simulink library "slrt2levelinverterlib"  (R2022b)
settings: Solver=VariableStepAuto  StartTime=0.0  StopTime=10.0  RelTol=1e-3
libraries: simulink x40, slrthdlutillib x12, hdlsllib x3
settings Model: Creator=chrisz  LastModifiedBy=chrisz
settings ModelReferenceCC: EnableRefExpFcnMdlSchedulingChecks=on
settings RTWCC: PlatformDefinition=Embedded Code

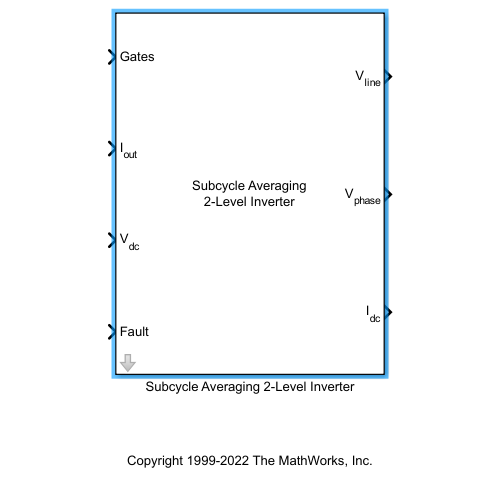
[thumbnail: Simulink's stored preview of the top-level diagram]
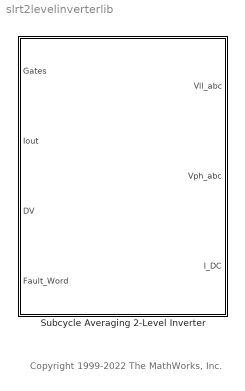
== system slrt2levelinverterlib ==
  note: Copyright 1999-2022 The MathWorks, Inc.
  "Subcycle Averaging 2-Level Inverter " : Subsystem  mask(Subcycle Averaging 2-level Inverter){rSwitch=0.1, vfSwitch=0.8, rDiode=0.2, vfDiode=0.6, rSnub=10000, ts_Model=1e-6, ts_FPGA=5e-9}
      mask prompts: rSwitch "Switch Resistance (Ohms)"; vfSwitch "Switch Forward Voltage (V)"; rDiode "Diode Resistance (Ohms)"; vfDiode "Diode Forward Voltage (V)"; rSnub "Snubber Resistance (Ohms)"; ts_Model "Model Time Step (s)"; ts_FPGA "FPGA Time Step (s)"
      mask help:
      | 2 level inverter with subcycle averaging that is meant for implementation of real-time models.  This model simulates FPGA clock level operations and is not suited for desktop simulation other than for validating the real-time model is accurate.  It should primarily be used when generating HDL for real-time systems. Use standard converter models and blocks for desktop simulation.
      |
      | Model time step should be 1/10 of switching frequency to capture accurate switching waveforms. FPGA time step should be the fastest time step you can run your HIL FPGA at.
      mask DialogControl ParameterGroupVar Prompt: Physical Parameters
      mask DialogControl Container3 Prompt: Simulation Parameters
      mask Display:
      | disp('Subcycle Averaging\n2-Level Inverter');
      | port_label('input',1,'Gates');
      | port_label('input',2,'I_o_u_t','texmode','on');
      | port_label('input',3,'V_d_c','texmode','on');
      | port_label('input',4,'Fault');
      | port_label('output',1,'V_l_i_n_e','texmode','on');
      | port_label('output',2,'V_p_h_a_s_e','texmode','on');
      | port_label('output',3,'I_d_c','texmode','on');

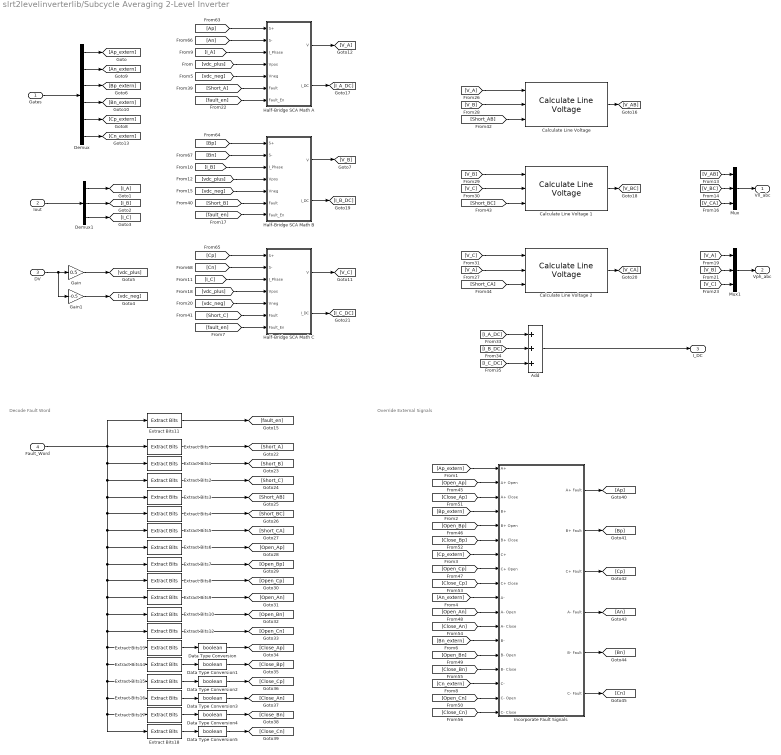
== system slrt2levelinverterlib/Subcycle Averaging 2-Level Inverter  ==
  note: Override External Signals
  note: Decode Fault Word
  Gates : Inport
  Iout : Inport  Port=2
  DV : Inport  Port=3
  Fault_Word : Inport  Port=4
  Add : Sum  Inputs=+++
  "Calculate Line Voltage " : slrthdlutillib/Calculate Line Voltage 
  Calculate Line Voltage 1 : slrthdlutillib/Calculate Line Voltage 
  Calculate Line Voltage 2 : slrthdlutillib/Calculate Line Voltage 
  Data Type Conversion{,1..5} (6 alike) : DataTypeConversion  OutDataTypeStr=boolean  SaturateOnIntegerOverflow=off  RndMeth=Floor
  Demux : Demux  Outputs=6
  Demux1 : Demux  Outputs=3
  Extract Bits : simulink/Logic and Bit Operations/Extract Bits  bitsToExtract=Range of bits  numBits=8  bitIdxRange=[0]  outScalingMode=Treat bit field as an integer
  Extract Bits1 : simulink/Logic and Bit Operations/Extract Bits  bitsToExtract=Range of bits  numBits=8  bitIdxRange=1  outScalingMode=Treat bit field as an integer
  Extract Bits10 : simulink/Logic and Bit Operations/Extract Bits  bitsToExtract=Range of bits  numBits=8  bitIdxRange=10  outScalingMode=Treat bit field as an integer
  Extract Bits11 : simulink/Logic and Bit Operations/Extract Bits  bitsToExtract=Range of bits  numBits=8  bitIdxRange=[31]  outScalingMode=Treat bit field as an integer
  Extract Bits12 : simulink/Logic and Bit Operations/Extract Bits  bitsToExtract=Range of bits  numBits=8  bitIdxRange=11  outScalingMode=Treat bit field as an integer
  Extract Bits13 : simulink/Logic and Bit Operations/Extract Bits  bitsToExtract=Range of bits  numBits=8  bitIdxRange=12  outScalingMode=Treat bit field as an integer
  Extract Bits14 : simulink/Logic and Bit Operations/Extract Bits  bitsToExtract=Range of bits  numBits=8  bitIdxRange=13  outScalingMode=Treat bit field as an integer
  Extract Bits15 : simulink/Logic and Bit Operations/Extract Bits  bitsToExtract=Range of bits  numBits=8  bitIdxRange=14  outScalingMode=Treat bit field as an integer
  Extract Bits16 : simulink/Logic and Bit Operations/Extract Bits  bitsToExtract=Range of bits  numBits=8  bitIdxRange=15  outScalingMode=Treat bit field as an integer
  Extract Bits17 : simulink/Logic and Bit Operations/Extract Bits  bitsToExtract=Range of bits  numBits=8  bitIdxRange=16  outScalingMode=Treat bit field as an integer
  Extract Bits18 : simulink/Logic and Bit Operations/Extract Bits  bitsToExtract=Range of bits  numBits=8  bitIdxRange=17  outScalingMode=Treat bit field as an integer
  Extract Bits2 : simulink/Logic and Bit Operations/Extract Bits  bitsToExtract=Range of bits  numBits=8  bitIdxRange=2  outScalingMode=Treat bit field as an integer
  Extract Bits3 : simulink/Logic and Bit Operations/Extract Bits  bitsToExtract=Range of bits  numBits=8  bitIdxRange=3  outScalingMode=Treat bit field as an integer
  Extract Bits4 : simulink/Logic and Bit Operations/Extract Bits  bitsToExtract=Range of bits  numBits=8  bitIdxRange=4  outScalingMode=Treat bit field as an integer
  Extract Bits5 : simulink/Logic and Bit Operations/Extract Bits  bitsToExtract=Range of bits  numBits=8  bitIdxRange=5  outScalingMode=Treat bit field as an integer
  Extract Bits6 : simulink/Logic and Bit Operations/Extract Bits  bitsToExtract=Range of bits  numBits=8  bitIdxRange=6  outScalingMode=Treat bit field as an integer
  Extract Bits7 : simulink/Logic and Bit Operations/Extract Bits  bitsToExtract=Range of bits  numBits=8  bitIdxRange=7  outScalingMode=Treat bit field as an integer
  Extract Bits8 : simulink/Logic and Bit Operations/Extract Bits  bitsToExtract=Range of bits  numBits=8  bitIdxRange=8  outScalingMode=Treat bit field as an integer
  Extract Bits9 : simulink/Logic and Bit Operations/Extract Bits  bitsToExtract=Range of bits  numBits=8  bitIdxRange=9  outScalingMode=Treat bit field as an integer
  Gain : Gain  Gain=0.5
  Gain1 : Gain  Gain=-0.5
  Half-Bridge SCA Math A : Subsystem
  Half-Bridge SCA Math B : Subsystem
  Half-Bridge SCA Math C : Subsystem
  Incorporate Fault Signals : Subsystem
  Mux : Mux  Inputs=3
  Mux1 : Mux  Inputs=3
  Vll_abc : Outport  OutDataTypeStr=single  VectorParamsAs1DForOutWhenUnconnected=off
  Vph_abc : Outport  Port=2  OutDataTypeStr=single  VectorParamsAs1DForOutWhenUnconnected=off
  I_DC : Outport  Port=3  OutDataTypeStr=single  VectorParamsAs1DForOutWhenUnconnected=off
  wires:
  Gates/1 -> Demux/1
  Demux/1 -> [Ap_extern]
  Demux/3 -> [Bp_extern]
  Demux/5 -> [Cp_extern]
  Half-Bridge SCA Math A/1(V) -> [V_A]
  [V_B] -> "Calculate Line Voltage "/2
  [V_A] -> "Calculate Line Voltage "/1
  Extract Bits9/1 -> [Open_An]
  Extract Bits12/1 -> [Open_Cn]
  [Ap_extern] -> Incorporate Fault Signals/1(A+)
  Incorporate Fault Signals/6(C- Fault) -> [Cn]
  [Open_Cn] -> Incorporate Fault Signals/17(C- Open)
  Incorporate Fault Signals/2(B+ Fault) -> [Bp]
  [Cn_extern] -> Incorporate Fault Signals/16(C-)
  [Close_Bn] -> Incorporate Fault Signals/15(B- Close)
  Incorporate Fault Signals/5(B- Fault) -> [Bn]
  Extract Bits7/1 -> [Open_Bp]
  [Bp_extern] -> Incorporate Fault Signals/4(B+)
  [Close_Cn] -> Incorporate Fault Signals/18(C- Close)
  [Close_Bp] -> Incorporate Fault Signals/6(B+ Close)
  [Open_Bp] -> Incorporate Fault Signals/5(B+ Open)
  [Bn_extern] -> Incorporate Fault Signals/13(B-)
  [Close_An] -> Incorporate Fault Signals/12(A- Close)
  [An_extern] -> Incorporate Fault Signals/10(A-)
  Fault_Word/1 -> Extract Bits11/1, Extract Bits/1, Extract Bits1/1, Extract Bits2/1, Extract Bits3/1, Extract Bits4/1, Extract Bits5/1, Extract Bits6/1, Extract Bits7/1, Extract Bits8/1, Extract Bits9/1, Extract Bits10/1, Extract Bits12/1, Extract Bits13/1, Extract Bits14/1, Extract Bits15/1, Extract Bits16/1, Extract Bits18/1, Extract Bits17/1
  Extract Bits6/1 -> [Open_Ap]
  [Open_Ap] -> Incorporate Fault Signals/2(A+ Open)
  Extract Bits8/1 -> [Open_Cp]
  Extract Bits17/1 -> Data Type Conversion4/1
  [Cp_extern] -> Incorporate Fault Signals/7(C+)
  Extract Bits5/1 -> [Short_CA]
  Extract Bits14/1 -> Data Type Conversion1/1
  Extract Bits1/1 -> [Short_B]
  Extract Bits13/1 -> Data Type Conversion/1
  Extract Bits10/1 -> [Open_Bn]
  Incorporate Fault Signals/4(A- Fault) -> [An]
  [Close_Ap] -> Incorporate Fault Signals/3(A+ Close)
  [Open_Cp] -> Incorporate Fault Signals/8(C+ Open)
  Incorporate Fault Signals/1(A+ Fault) -> [Ap]
  Extract Bits4/1 -> [Short_BC]
  Extract Bits18/1 -> Data Type Conversion5/1
  Extract Bits3/1 -> [Short_AB]
  [Open_Bn] -> Incorporate Fault Signals/14(B- Open)
  Extract Bits2/1 -> [Short_C]
  [Open_An] -> Incorporate Fault Signals/11(A- Open)
  Extract Bits15/1 -> Data Type Conversion2/1
  Extract Bits/1 -> [Short_A]
  Incorporate Fault Signals/3(C+ Fault) -> [Cp]
  [Close_Cp] -> Incorporate Fault Signals/9(C+ Close)
  Extract Bits16/1 -> Data Type Conversion3/1
  Iout/1 -> Demux1/1
  Demux1/1 -> [I_A]
  Demux1/2 -> [I_B]
  Demux1/3 -> [I_C]
  [Ap] -> Half-Bridge SCA Math A/1(S+)
  [I_A] -> Half-Bridge SCA Math A/3(I_Phase)
  [An] -> Half-Bridge SCA Math A/2(S-)
  [vdc_plus] -> Half-Bridge SCA Math A/4(Vpos)
  [vdc_neg] -> Half-Bridge SCA Math A/5(Vneg)
  [Short_A] -> Half-Bridge SCA Math A/6(Fault)
  [Bp] -> Half-Bridge SCA Math B/1(S+)
  [Bn] -> Half-Bridge SCA Math B/2(S-)
  [I_B] -> Half-Bridge SCA Math B/3(I_Phase)
  [vdc_plus] -> Half-Bridge SCA Math B/4(Vpos)
  [vdc_neg] -> Half-Bridge SCA Math B/5(Vneg)
  [Short_B] -> Half-Bridge SCA Math B/6(Fault)
  [I_C] -> Half-Bridge SCA Math C/3(I_Phase)
  [Cp] -> Half-Bridge SCA Math C/1(S+)
  [Cn] -> Half-Bridge SCA Math C/2(S-)
  [vdc_plus] -> Half-Bridge SCA Math C/4(Vpos)
  [vdc_neg] -> Half-Bridge SCA Math C/5(Vneg)
  [Short_C] -> Half-Bridge SCA Math C/6(Fault)
  Half-Bridge SCA Math B/1(V) -> [V_B]
  Half-Bridge SCA Math C/1(V) -> [V_C]
  [V_C] -> Calculate Line Voltage 2/1
  [V_A] -> Calculate Line Voltage 2/2
  [V_C] -> Calculate Line Voltage 1/2
  [Short_AB] -> "Calculate Line Voltage "/3
  [Short_BC] -> Calculate Line Voltage 1/3
  [Short_CA] -> Calculate Line Voltage 2/3
  [V_BC] -> Mux/2
  [V_CA] -> Mux/3
  [V_AB] -> Mux/1
  Mux/1 -> Vll_abc/1
  Data Type Conversion/1 -> [Close_Ap]
  Data Type Conversion1/1 -> [Close_Bp]
  Data Type Conversion2/1 -> [Close_Cp]
  Data Type Conversion3/1 -> [Close_An]
  Data Type Conversion4/1 -> [Close_Bn]
  Data Type Conversion5/1 -> [Close_Cn]
  Mux1/1 -> Vph_abc/1
  [V_A] -> Mux1/1
  [V_C] -> Mux1/3
  [V_B] -> Mux1/2
  Demux/2 -> [An_extern]
  Demux/4 -> [Bn_extern]
  Demux/6 -> [Cn_extern]
  Half-Bridge SCA Math A/2(I_DC) -> [I_A_DC]
  Half-Bridge SCA Math B/2(I_DC) -> [I_B_DC]
  Half-Bridge SCA Math C/2(I_DC) -> [I_C_DC]
  [I_A_DC] -> Add/1
  [I_B_DC] -> Add/2
  [I_C_DC] -> Add/3
  Add/1 -> I_DC/1
  Extract Bits11/1 -> [fault_en]
  [fault_en] -> Half-Bridge SCA Math A/7(Fault_En)
  [fault_en] -> Half-Bridge SCA Math B/7(Fault_En)
  [fault_en] -> Half-Bridge SCA Math C/7(Fault_En)
  "Calculate Line Voltage "/1 -> [V_AB]
  Calculate Line Voltage 1/1 -> [V_BC]
  [V_B] -> Calculate Line Voltage 1/1
  Calculate Line Voltage 2/1 -> [V_CA]
  DV/1 -> Gain1/1, Gain/1
  Gain/1 -> [vdc_plus]
  Gain1/1 -> [vdc_neg]

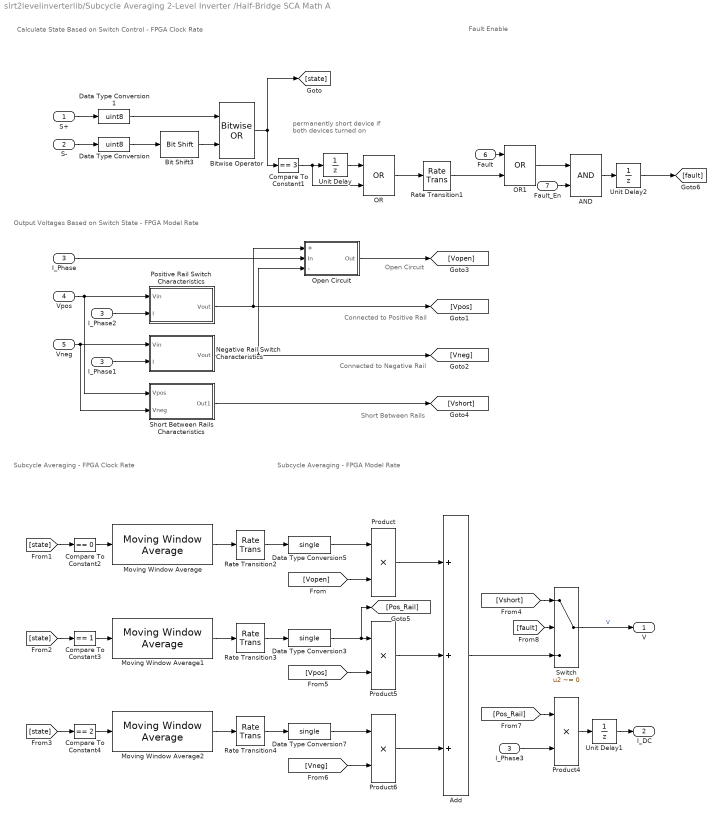
== system slrt2levelinverterlib/Subcycle Averaging 2-Level Inverter /Half-Bridge SCA Math A ==
  note: permanently short device if both devices turned on
  note: Subcycle Averaging - FPGA Clock Rate
  note: Open Circuit
  note: Connected to Positive Rail
  note: Connected to Negative Rail
  note: Short Between Rails
  note: Subcycle Averaging - FPGA Model Rate
  note: Output Voltages Based on Switch State - FPGA Model Rate
  note: Calculate State Based on Switch Control - FPGA Clock Rate
  note: Fault Enable
  S+ : Inport
  S- : Inport  Port=2
  I_Phase : Inport  Port=3
  Vpos : Inport  Port=4
  Vneg : Inport  Port=5
  Fault : Inport  Port=6
  Fault_En : Inport  Port=7
  AND : Logic  IconShape=distinctive  AllPortsSameDT=off  OutDataTypeStr=boolean
  Add : Sum  Inputs=+++
  Bit Shift3 : hdlsllib/Logic and Bit Operations/Bit Shift  mode=Shift Left Logical  N=1
  Bitwise Operator : simulink/Logic and Bit Operations/Bitwise Operator  logicop=OR  UseBitMask=off  NumInputPorts=2  BitMask=bin2dec('11011001')  BitMaskRealWorld=Stored Integer
  Compare To Constant1 : simulink/Logic and Bit Operations/Compare To Constant  relop===  const=3  OutDataTypeStr=boolean
  Compare To Constant2 : simulink/Logic and Bit Operations/Compare To Constant  relop===  const=0  OutDataTypeStr=boolean
  Compare To Constant3 : simulink/Logic and Bit Operations/Compare To Constant  relop===  const=1  OutDataTypeStr=boolean
  Compare To Constant4 : simulink/Logic and Bit Operations/Compare To Constant  relop===  const=2  OutDataTypeStr=boolean
  Data Type Conversion : DataTypeConversion  OutDataTypeStr=uint8  SaturateOnIntegerOverflow=off  RndMeth=Floor
  Data Type Conversion1 : DataTypeConversion  OutDataTypeStr=uint8  SaturateOnIntegerOverflow=off  RndMeth=Floor
  Data Type Conversion3 : DataTypeConversion  OutDataTypeStr=single  SaturateOnIntegerOverflow=off  RndMeth=Floor
  Data Type Conversion5 : DataTypeConversion  OutDataTypeStr=single  SaturateOnIntegerOverflow=off  RndMeth=Floor
  Data Type Conversion7 : DataTypeConversion  OutDataTypeStr=single  SaturateOnIntegerOverflow=off  RndMeth=Floor
  I_Phase1 : InportShadow  Port=3
  I_Phase2 : InportShadow  Port=3
  I_Phase3 : InportShadow  Port=3
  Moving Window Average : slrthdlutillib/Moving Window Average  sample_time=ts_FPGA  window_size=ts_Model
  Moving Window Average1 : slrthdlutillib/Moving Window Average  sample_time=ts_FPGA  window_size=ts_Model
  Moving Window Average2 : slrthdlutillib/Moving Window Average  sample_time=ts_FPGA  window_size=ts_Model
  Negative Rail Switch Characteristics : Subsystem
  OR : Logic  Operator=OR  IconShape=distinctive  AllPortsSameDT=off  OutDataTypeStr=boolean
  OR1 : Logic  Operator=OR  IconShape=distinctive  AllPortsSameDT=off  OutDataTypeStr=boolean
  Open Circuit : Subsystem
  Positive Rail Switch Characteristics : Subsystem
  Product{,4..6} (4 alike) : Product
  Rate Transition{1..4} (4 alike) : RateTransition  OutPortSampleTime=ts_Model
  Short Between Rails Characteristics : Subsystem
  Switch : Switch  Criteria=u2 ~= 0  SaturateOnIntegerOverflow=off  InputSameDT=off
  Unit Delay : UnitDelay  SampleTime=-1  HasFrameUpgradeWarning=on
  Unit Delay1 : UnitDelay  SampleTime=-1  HasFrameUpgradeWarning=on
  Unit Delay2 : UnitDelay  SampleTime=-1  HasFrameUpgradeWarning=on
  V : Outport  VectorParamsAs1DForOutWhenUnconnected=off
  I_DC : Outport  Port=2  VectorParamsAs1DForOutWhenUnconnected=off
  wires:
  Unit Delay2/1 -> [fault]
  Switch/1 -> V/1  "V"
  Bit Shift3/1 -> Bitwise Operator/2
  Vpos/1 -> Short Between Rails Characteristics/1(Vpos), Positive Rail Switch Characteristics/1(Vin)
  Open Circuit/1(Out) -> [Vopen]
  Data Type Conversion/1 -> Bit Shift3/1
  Data Type Conversion1/1 -> Bitwise Operator/1
  Vneg/1 -> Short Between Rails Characteristics/2(Vneg), Negative Rail Switch Characteristics/1(Vin)
  I_Phase/1 -> Open Circuit/2(In)
  [fault] -> Switch/2
  Negative Rail Switch Characteristics/1(Vout) -> [Vneg], Open Circuit/3(-)
  Positive Rail Switch Characteristics/1(Vout) -> [Vpos], Open Circuit/1(+)
  I_Phase2/1 -> Positive Rail Switch Characteristics/2(I)
  I_Phase1/1 -> Negative Rail Switch Characteristics/2(I)
  S-/1 -> Data Type Conversion/1
  Moving Window Average/1 -> Rate Transition2/1
  S+/1 -> Data Type Conversion1/1
  Bitwise Operator/1 -> [state], Compare To Constant1/1
  [state] -> Compare To Constant3/1
  [state] -> Compare To Constant2/1
  [state] -> Compare To Constant4/1
  Moving Window Average1/1 -> Rate Transition3/1
  Moving Window Average2/1 -> Rate Transition4/1
  Add/1 -> Switch/3
  Data Type Conversion5/1 -> Product/1
  [Vopen] -> Product/2
  Data Type Conversion3/1 -> [Pos_Rail], Product5/1
  [Vpos] -> Product5/2
  Data Type Conversion7/1 -> Product6/1
  [Vneg] -> Product6/2
  Product/1 -> Add/1
  Product5/1 -> Add/2
  Product6/1 -> Add/3
  Product4/1 -> Unit Delay1/1
  I_Phase3/1 -> Product4/2
  [Pos_Rail] -> Product4/1
  Unit Delay1/1 -> I_DC/1
  Compare To Constant2/1 -> Moving Window Average/1
  Compare To Constant4/1 -> Moving Window Average2/1
  Compare To Constant3/1 -> Moving Window Average1/1
  [Vshort] -> Switch/1
  Compare To Constant1/1 -> OR/2, Unit Delay/1
  Unit Delay/1 -> OR/1
  OR/1 -> Rate Transition1/1
  Fault/1 -> OR1/1
  OR1/1 -> AND/1
  Rate Transition1/1 -> OR1/2
  AND/1 -> Unit Delay2/1
  Fault_En/1 -> AND/2
  Rate Transition2/1 -> Data Type Conversion5/1
  Rate Transition3/1 -> Data Type Conversion3/1
  Rate Transition4/1 -> Data Type Conversion7/1
  Short Between Rails Characteristics/1(Out1) -> [Vshort]

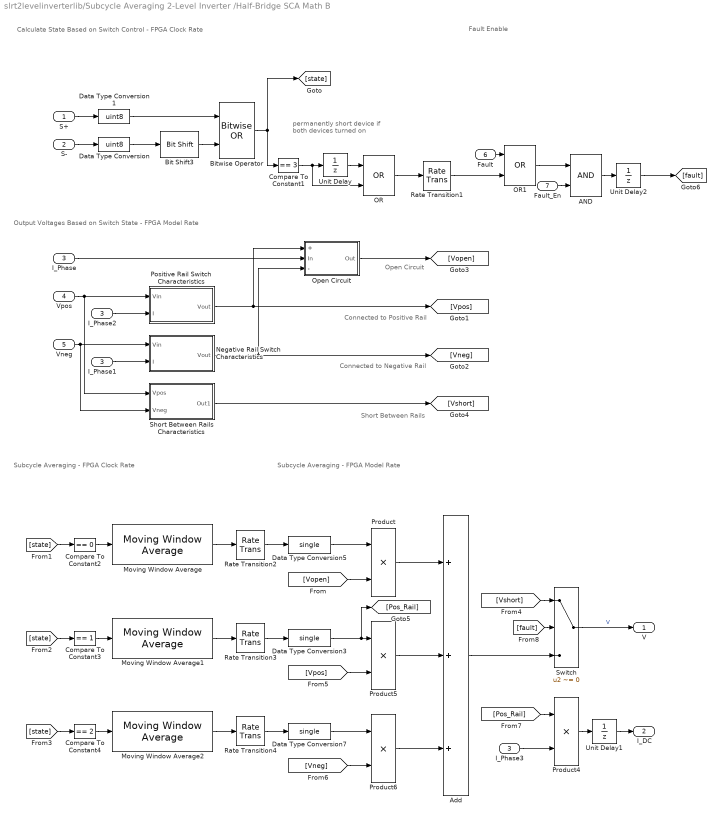
== system slrt2levelinverterlib/Subcycle Averaging 2-Level Inverter /Half-Bridge SCA Math B ==
  note: permanently short device if both devices turned on
  note: Subcycle Averaging - FPGA Clock Rate
  note: Open Circuit
  note: Connected to Positive Rail
  note: Connected to Negative Rail
  note: Short Between Rails
  note: Subcycle Averaging - FPGA Model Rate
  note: Output Voltages Based on Switch State - FPGA Model Rate
  note: Calculate State Based on Switch Control - FPGA Clock Rate
  note: Fault Enable
  S+ : Inport
  S- : Inport  Port=2
  I_Phase : Inport  Port=3
  Vpos : Inport  Port=4
  Vneg : Inport  Port=5
  Fault : Inport  Port=6
  Fault_En : Inport  Port=7
  AND : Logic  IconShape=distinctive  AllPortsSameDT=off  OutDataTypeStr=boolean
  Add : Sum  Inputs=+++
  Bit Shift3 : hdlsllib/Logic and Bit Operations/Bit Shift  mode=Shift Left Logical  N=1
  Bitwise Operator : simulink/Logic and Bit Operations/Bitwise Operator  logicop=OR  UseBitMask=off  NumInputPorts=2  BitMask=bin2dec('11011001')  BitMaskRealWorld=Stored Integer
  Compare To Constant1 : simulink/Logic and Bit Operations/Compare To Constant  relop===  const=3  OutDataTypeStr=boolean
  Compare To Constant2 : simulink/Logic and Bit Operations/Compare To Constant  relop===  const=0  OutDataTypeStr=boolean
  Compare To Constant3 : simulink/Logic and Bit Operations/Compare To Constant  relop===  const=1  OutDataTypeStr=boolean
  Compare To Constant4 : simulink/Logic and Bit Operations/Compare To Constant  relop===  const=2  OutDataTypeStr=boolean
  Data Type Conversion : DataTypeConversion  OutDataTypeStr=uint8  SaturateOnIntegerOverflow=off  RndMeth=Floor
  Data Type Conversion1 : DataTypeConversion  OutDataTypeStr=uint8  SaturateOnIntegerOverflow=off  RndMeth=Floor
  Data Type Conversion3 : DataTypeConversion  OutDataTypeStr=single  SaturateOnIntegerOverflow=off  RndMeth=Floor
  Data Type Conversion5 : DataTypeConversion  OutDataTypeStr=single  SaturateOnIntegerOverflow=off  RndMeth=Floor
  Data Type Conversion7 : DataTypeConversion  OutDataTypeStr=single  SaturateOnIntegerOverflow=off  RndMeth=Floor
  I_Phase1 : InportShadow  Port=3
  I_Phase2 : InportShadow  Port=3
  I_Phase3 : InportShadow  Port=3
  Moving Window Average : slrthdlutillib/Moving Window Average  sample_time=ts_FPGA  window_size=ts_Model
  Moving Window Average1 : slrthdlutillib/Moving Window Average  sample_time=ts_FPGA  window_size=ts_Model
  Moving Window Average2 : slrthdlutillib/Moving Window Average  sample_time=ts_FPGA  window_size=ts_Model
  Negative Rail Switch Characteristics : Subsystem
  OR : Logic  Operator=OR  IconShape=distinctive  AllPortsSameDT=off  OutDataTypeStr=boolean
  OR1 : Logic  Operator=OR  IconShape=distinctive  AllPortsSameDT=off  OutDataTypeStr=boolean
  Open Circuit : Subsystem
  Positive Rail Switch Characteristics : Subsystem
  Product{,4..6} (4 alike) : Product
  Rate Transition{1..4} (4 alike) : RateTransition  OutPortSampleTime=ts_Model
  Short Between Rails Characteristics : Subsystem
  Switch : Switch  Criteria=u2 ~= 0  SaturateOnIntegerOverflow=off  InputSameDT=off
  Unit Delay : UnitDelay  SampleTime=-1  HasFrameUpgradeWarning=on
  Unit Delay1 : UnitDelay  SampleTime=-1  HasFrameUpgradeWarning=on
  Unit Delay2 : UnitDelay  SampleTime=-1  HasFrameUpgradeWarning=on
  V : Outport  VectorParamsAs1DForOutWhenUnconnected=off
  I_DC : Outport  Port=2  VectorParamsAs1DForOutWhenUnconnected=off
  wires:
  Unit Delay2/1 -> [fault]
  Switch/1 -> V/1  "V"
  Bit Shift3/1 -> Bitwise Operator/2
  Vpos/1 -> Short Between Rails Characteristics/1(Vpos), Positive Rail Switch Characteristics/1(Vin)
  Open Circuit/1(Out) -> [Vopen]
  Data Type Conversion/1 -> Bit Shift3/1
  Data Type Conversion1/1 -> Bitwise Operator/1
  Vneg/1 -> Short Between Rails Characteristics/2(Vneg), Negative Rail Switch Characteristics/1(Vin)
  I_Phase/1 -> Open Circuit/2(In)
  [fault] -> Switch/2
  Negative Rail Switch Characteristics/1(Vout) -> [Vneg], Open Circuit/3(-)
  Positive Rail Switch Characteristics/1(Vout) -> [Vpos], Open Circuit/1(+)
  I_Phase2/1 -> Positive Rail Switch Characteristics/2(I)
  I_Phase1/1 -> Negative Rail Switch Characteristics/2(I)
  S-/1 -> Data Type Conversion/1
  Moving Window Average/1 -> Rate Transition2/1
  S+/1 -> Data Type Conversion1/1
  Bitwise Operator/1 -> [state], Compare To Constant1/1
  [state] -> Compare To Constant3/1
  [state] -> Compare To Constant2/1
  [state] -> Compare To Constant4/1
  Moving Window Average1/1 -> Rate Transition3/1
  Moving Window Average2/1 -> Rate Transition4/1
  Add/1 -> Switch/3
  Data Type Conversion5/1 -> Product/1
  [Vopen] -> Product/2
  Data Type Conversion3/1 -> [Pos_Rail], Product5/1
  [Vpos] -> Product5/2
  Data Type Conversion7/1 -> Product6/1
  [Vneg] -> Product6/2
  Product/1 -> Add/1
  Product5/1 -> Add/2
  Product6/1 -> Add/3
  Product4/1 -> Unit Delay1/1
  I_Phase3/1 -> Product4/2
  [Pos_Rail] -> Product4/1
  Unit Delay1/1 -> I_DC/1
  Compare To Constant2/1 -> Moving Window Average/1
  Compare To Constant4/1 -> Moving Window Average2/1
  Compare To Constant3/1 -> Moving Window Average1/1
  [Vshort] -> Switch/1
  Compare To Constant1/1 -> OR/2, Unit Delay/1
  Unit Delay/1 -> OR/1
  OR/1 -> Rate Transition1/1
  Fault/1 -> OR1/1
  OR1/1 -> AND/1
  Rate Transition1/1 -> OR1/2
  AND/1 -> Unit Delay2/1
  Fault_En/1 -> AND/2
  Rate Transition2/1 -> Data Type Conversion5/1
  Rate Transition3/1 -> Data Type Conversion3/1
  Rate Transition4/1 -> Data Type Conversion7/1
  Short Between Rails Characteristics/1(Out1) -> [Vshort]

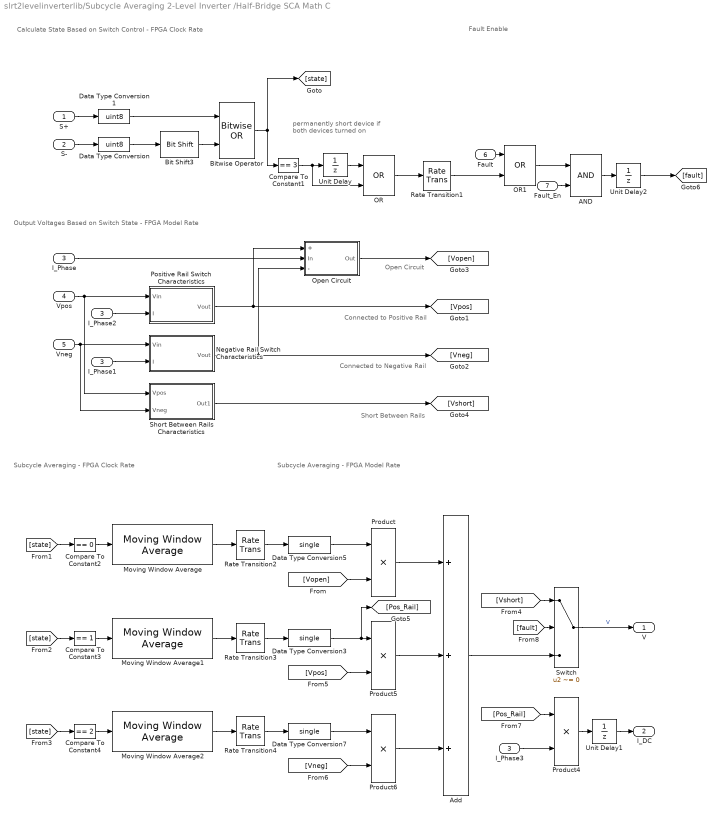
== system slrt2levelinverterlib/Subcycle Averaging 2-Level Inverter /Half-Bridge SCA Math C ==
  note: permanently short device if both devices turned on
  note: Subcycle Averaging - FPGA Clock Rate
  note: Open Circuit
  note: Connected to Positive Rail
  note: Connected to Negative Rail
  note: Short Between Rails
  note: Subcycle Averaging - FPGA Model Rate
  note: Output Voltages Based on Switch State - FPGA Model Rate
  note: Calculate State Based on Switch Control - FPGA Clock Rate
  note: Fault Enable
  S+ : Inport
  S- : Inport  Port=2
  I_Phase : Inport  Port=3
  Vpos : Inport  Port=4
  Vneg : Inport  Port=5
  Fault : Inport  Port=6
  Fault_En : Inport  Port=7
  AND : Logic  IconShape=distinctive  AllPortsSameDT=off  OutDataTypeStr=boolean
  Add : Sum  Inputs=+++
  Bit Shift3 : hdlsllib/Logic and Bit Operations/Bit Shift  mode=Shift Left Logical  N=1
  Bitwise Operator : simulink/Logic and Bit Operations/Bitwise Operator  logicop=OR  UseBitMask=off  NumInputPorts=2  BitMask=bin2dec('11011001')  BitMaskRealWorld=Stored Integer
  Compare To Constant1 : simulink/Logic and Bit Operations/Compare To Constant  relop===  const=3  OutDataTypeStr=boolean
  Compare To Constant2 : simulink/Logic and Bit Operations/Compare To Constant  relop===  const=0  OutDataTypeStr=boolean
  Compare To Constant3 : simulink/Logic and Bit Operations/Compare To Constant  relop===  const=1  OutDataTypeStr=boolean
  Compare To Constant4 : simulink/Logic and Bit Operations/Compare To Constant  relop===  const=2  OutDataTypeStr=boolean
  Data Type Conversion : DataTypeConversion  OutDataTypeStr=uint8  SaturateOnIntegerOverflow=off  RndMeth=Floor
  Data Type Conversion1 : DataTypeConversion  OutDataTypeStr=uint8  SaturateOnIntegerOverflow=off  RndMeth=Floor
  Data Type Conversion3 : DataTypeConversion  OutDataTypeStr=single  SaturateOnIntegerOverflow=off  RndMeth=Floor
  Data Type Conversion5 : DataTypeConversion  OutDataTypeStr=single  SaturateOnIntegerOverflow=off  RndMeth=Floor
  Data Type Conversion7 : DataTypeConversion  OutDataTypeStr=single  SaturateOnIntegerOverflow=off  RndMeth=Floor
  I_Phase1 : InportShadow  Port=3
  I_Phase2 : InportShadow  Port=3
  I_Phase3 : InportShadow  Port=3
  Moving Window Average : slrthdlutillib/Moving Window Average  sample_time=ts_FPGA  window_size=ts_Model
  Moving Window Average1 : slrthdlutillib/Moving Window Average  sample_time=ts_FPGA  window_size=ts_Model
  Moving Window Average2 : slrthdlutillib/Moving Window Average  sample_time=ts_FPGA  window_size=ts_Model
  Negative Rail Switch Characteristics : Subsystem
  OR : Logic  Operator=OR  IconShape=distinctive  AllPortsSameDT=off  OutDataTypeStr=boolean
  OR1 : Logic  Operator=OR  IconShape=distinctive  AllPortsSameDT=off  OutDataTypeStr=boolean
  Open Circuit : Subsystem
  Positive Rail Switch Characteristics : Subsystem
  Product{,4..6} (4 alike) : Product
  Rate Transition{1..4} (4 alike) : RateTransition  OutPortSampleTime=ts_Model
  Short Between Rails Characteristics : Subsystem
  Switch : Switch  Criteria=u2 ~= 0  SaturateOnIntegerOverflow=off  InputSameDT=off
  Unit Delay : UnitDelay  SampleTime=-1  HasFrameUpgradeWarning=on
  Unit Delay1 : UnitDelay  SampleTime=-1  HasFrameUpgradeWarning=on
  Unit Delay2 : UnitDelay  SampleTime=-1  HasFrameUpgradeWarning=on
  V : Outport  VectorParamsAs1DForOutWhenUnconnected=off
  I_DC : Outport  Port=2  VectorParamsAs1DForOutWhenUnconnected=off
  wires:
  Unit Delay2/1 -> [fault]
  Switch/1 -> V/1  "V"
  Bit Shift3/1 -> Bitwise Operator/2
  Vpos/1 -> Short Between Rails Characteristics/1(Vpos), Positive Rail Switch Characteristics/1(Vin)
  Open Circuit/1(Out) -> [Vopen]
  Data Type Conversion/1 -> Bit Shift3/1
  Data Type Conversion1/1 -> Bitwise Operator/1
  Vneg/1 -> Short Between Rails Characteristics/2(Vneg), Negative Rail Switch Characteristics/1(Vin)
  I_Phase/1 -> Open Circuit/2(In)
  [fault] -> Switch/2
  Negative Rail Switch Characteristics/1(Vout) -> [Vneg], Open Circuit/3(-)
  Positive Rail Switch Characteristics/1(Vout) -> [Vpos], Open Circuit/1(+)
  I_Phase2/1 -> Positive Rail Switch Characteristics/2(I)
  I_Phase1/1 -> Negative Rail Switch Characteristics/2(I)
  S-/1 -> Data Type Conversion/1
  Moving Window Average/1 -> Rate Transition2/1
  S+/1 -> Data Type Conversion1/1
  Bitwise Operator/1 -> [state], Compare To Constant1/1
  [state] -> Compare To Constant3/1
  [state] -> Compare To Constant2/1
  [state] -> Compare To Constant4/1
  Moving Window Average1/1 -> Rate Transition3/1
  Moving Window Average2/1 -> Rate Transition4/1
  Add/1 -> Switch/3
  Data Type Conversion5/1 -> Product/1
  [Vopen] -> Product/2
  Data Type Conversion3/1 -> [Pos_Rail], Product5/1
  [Vpos] -> Product5/2
  Data Type Conversion7/1 -> Product6/1
  [Vneg] -> Product6/2
  Product/1 -> Add/1
  Product5/1 -> Add/2
  Product6/1 -> Add/3
  Product4/1 -> Unit Delay1/1
  I_Phase3/1 -> Product4/2
  [Pos_Rail] -> Product4/1
  Unit Delay1/1 -> I_DC/1
  Compare To Constant2/1 -> Moving Window Average/1
  Compare To Constant4/1 -> Moving Window Average2/1
  Compare To Constant3/1 -> Moving Window Average1/1
  [Vshort] -> Switch/1
  Compare To Constant1/1 -> OR/2, Unit Delay/1
  Unit Delay/1 -> OR/1
  OR/1 -> Rate Transition1/1
  Fault/1 -> OR1/1
  OR1/1 -> AND/1
  Rate Transition1/1 -> OR1/2
  AND/1 -> Unit Delay2/1
  Fault_En/1 -> AND/2
  Rate Transition2/1 -> Data Type Conversion5/1
  Rate Transition3/1 -> Data Type Conversion3/1
  Rate Transition4/1 -> Data Type Conversion7/1
  Short Between Rails Characteristics/1(Out1) -> [Vshort]

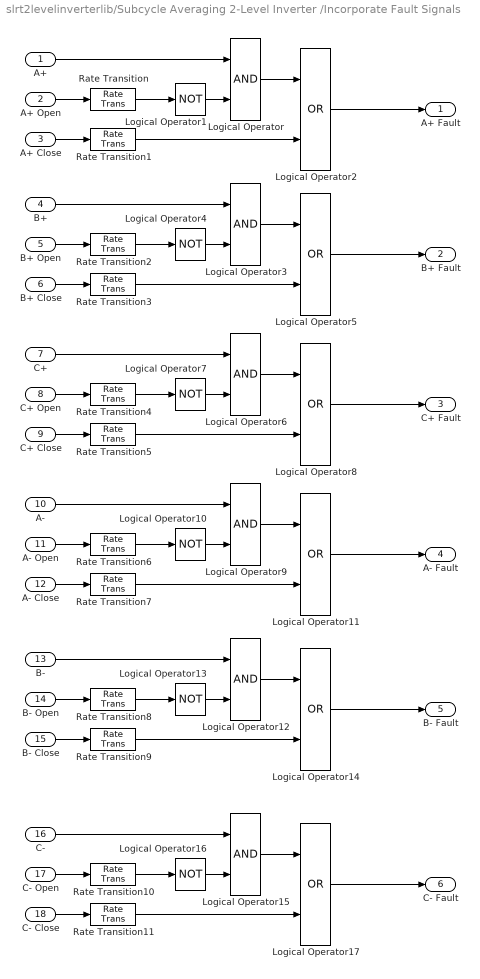
== system slrt2levelinverterlib/Subcycle Averaging 2-Level Inverter /Incorporate Fault Signals ==
  A+ : Inport
  A+ Open : Inport  Port=2
  A+ Close : Inport  Port=3
  B+ : Inport  Port=4
  B+ Open : Inport  Port=5
  B+ Close : Inport  Port=6
  C+ : Inport  Port=7
  C+ Open : Inport  Port=8
  C+ Close : Inport  Port=9
  A- : Inport  Port=10
  A- Open : Inport  Port=11
  A- Close : Inport  Port=12
  B- : Inport  Port=13
  B- Open : Inport  Port=14
  B- Close : Inport  Port=15
  C- : Inport  Port=16
  C- Open : Inport  Port=17
  C- Close : Inport  Port=18
  Logical Operator{,3,6,9,12,15} (6 alike) : Logic  AllPortsSameDT=off  OutDataTypeStr=boolean
  Logical Operator{1,4,7,10,13,16} (6 alike) : Logic  Operator=NOT  AllPortsSameDT=off  OutDataTypeStr=boolean
  Logical Operator{2,5,8,11,14,17} (6 alike) : Logic  Operator=OR  AllPortsSameDT=off  OutDataTypeStr=boolean
  Rate Transition{,1..11} (12 alike) : RateTransition
  A+ Fault : Outport  VectorParamsAs1DForOutWhenUnconnected=off
  B+ Fault : Outport  Port=2  VectorParamsAs1DForOutWhenUnconnected=off
  C+ Fault : Outport  Port=3  VectorParamsAs1DForOutWhenUnconnected=off
  A- Fault : Outport  Port=4  VectorParamsAs1DForOutWhenUnconnected=off
  B- Fault : Outport  Port=5  VectorParamsAs1DForOutWhenUnconnected=off
  C- Fault : Outport  Port=6  VectorParamsAs1DForOutWhenUnconnected=off
  wires:
  Logical Operator1/1 -> Logical Operator/2
  A+ Open/1 -> Rate Transition/1
  A+ Close/1 -> Rate Transition1/1
  Logical Operator/1 -> Logical Operator2/1
  Logical Operator2/1 -> A+ Fault/1
  Logical Operator5/1 -> B+ Fault/1
  Logical Operator3/1 -> Logical Operator5/1
  B+ Close/1 -> Rate Transition3/1
  B+ Open/1 -> Rate Transition2/1
  Logical Operator4/1 -> Logical Operator3/2
  Logical Operator7/1 -> Logical Operator6/2
  C+ Close/1 -> Rate Transition5/1
  Logical Operator6/1 -> Logical Operator8/1
  Logical Operator8/1 -> C+ Fault/1
  Logical Operator11/1 -> A- Fault/1
  Logical Operator9/1 -> Logical Operator11/1
  A- Close/1 -> Rate Transition7/1
  Logical Operator10/1 -> Logical Operator9/2
  Logical Operator14/1 -> B- Fault/1
  Logical Operator12/1 -> Logical Operator14/1
  Logical Operator13/1 -> Logical Operator12/2
  B- Close/1 -> Rate Transition9/1
  Logical Operator17/1 -> C- Fault/1
  Logical Operator15/1 -> Logical Operator17/1
  Logical Operator16/1 -> Logical Operator15/2
  C- Close/1 -> Rate Transition11/1
  A- Open/1 -> Rate Transition6/1
  B- Open/1 -> Rate Transition8/1
  C- Open/1 -> Rate Transition10/1
  C+ Open/1 -> Rate Transition4/1
  A+/1 -> Logical Operator/1
  B+/1 -> Logical Operator3/1
  C+/1 -> Logical Operator6/1
  A-/1 -> Logical Operator9/1
  B-/1 -> Logical Operator12/1
  C-/1 -> Logical Operator15/1
  Rate Transition/1 -> Logical Operator1/1
  Rate Transition1/1 -> Logical Operator2/2
  Rate Transition2/1 -> Logical Operator4/1
  Rate Transition3/1 -> Logical Operator5/2
  Rate Transition4/1 -> Logical Operator7/1
  Rate Transition5/1 -> Logical Operator8/2
  Rate Transition6/1 -> Logical Operator10/1
  Rate Transition7/1 -> Logical Operator11/2
  Rate Transition8/1 -> Logical Operator13/1
  Rate Transition9/1 -> Logical Operator14/2
  Rate Transition10/1 -> Logical Operator16/1
  Rate Transition11/1 -> Logical Operator17/2

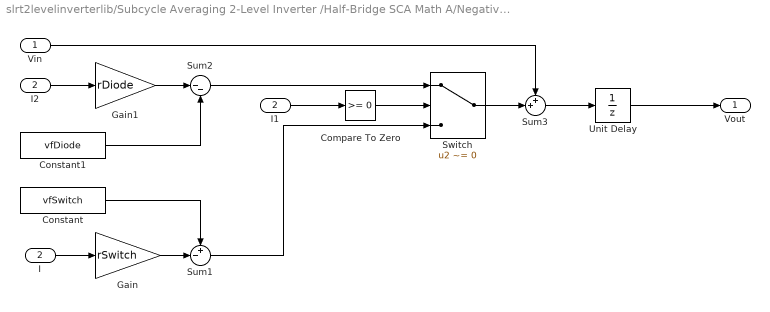
== system slrt2levelinverterlib/Subcycle Averaging 2-Level Inverter /Half-Bridge SCA Math A/Negative Rail Switch Characteristics ==
  Vin : Inport
  I : Inport  Port=2
  Compare To Zero : simulink/Logic and Bit Operations/Compare To Zero  relop=>=  OutDataTypeStr=boolean
  Constant : Constant  Value=vfSwitch  OutDataTypeStr=single  SampleTime=ts_Model
  Constant1 : Constant  Value=vfDiode  OutDataTypeStr=single  SampleTime=ts_Model
  Gain : Gain  Gain=rSwitch
  Gain1 : Gain  Gain=rDiode
  I1 : InportShadow  Port=2
  I2 : InportShadow  Port=2
  Sum1 : Sum  Inputs=+-|
  Sum2 : Sum  Inputs=|--
  Sum3 : Sum  Inputs=++|
  Switch : Switch  Criteria=u2 ~= 0  SaturateOnIntegerOverflow=off  InputSameDT=off
  Unit Delay : UnitDelay  SampleTime=-1  HasFrameUpgradeWarning=on
  Vout : Outport  VectorParamsAs1DForOutWhenUnconnected=off
  wires:
  I/1 -> Gain/1
  Gain1/1 -> Sum2/1
  Sum3/1 -> Unit Delay/1
  Switch/1 -> Sum3/2
  I1/1 -> Compare To Zero/1
  Vin/1 -> Sum3/1
  Unit Delay/1 -> Vout/1
  Constant/1 -> Sum1/1
  I2/1 -> Gain1/1
  Sum1/1 -> Switch/3
  Gain/1 -> Sum1/2
  Sum2/1 -> Switch/1
  Constant1/1 -> Sum2/2
  Compare To Zero/1 -> Switch/2

== system slrt2levelinverterlib/Subcycle Averaging 2-Level Inverter /Half-Bridge SCA Math A/Open Circuit ==
  + : Inport
  In : Inport  Port=2
  - : Inport  Port=3
  Gain : Gain  Gain=-rSnub
  Max : MinMax  Inputs=2
  Max1 : MinMax  Function=max  Inputs=2
  Unit Delay : UnitDelay  SampleTime=-1  HasFrameUpgradeWarning=on
  Out : Outport  VectorParamsAs1DForOutWhenUnconnected=off
  wires:
  -/1 -> Max1/2
  Max/1 -> Unit Delay/1
  +/1 -> Max/1
  Gain/1 -> Max1/1
  In/1 -> Gain/1
  Max1/1 -> Max/2
  Unit Delay/1 -> Out/1

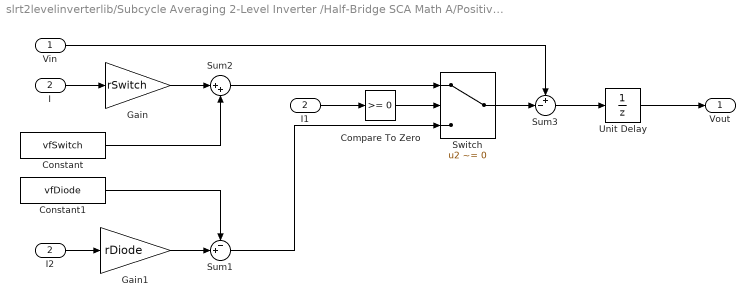
== system slrt2levelinverterlib/Subcycle Averaging 2-Level Inverter /Half-Bridge SCA Math A/Positive Rail Switch Characteristics ==
  Vin : Inport
  I : Inport  Port=2
  Compare To Zero : simulink/Logic and Bit Operations/Compare To Zero  relop=>=  OutDataTypeStr=boolean
  Constant : Constant  Value=vfSwitch  OutDataTypeStr=single  SampleTime=ts_Model
  Constant1 : Constant  Value=vfDiode  OutDataTypeStr=single  SampleTime=ts_Model
  Gain : Gain  Gain=rSwitch
  Gain1 : Gain  Gain=rDiode
  I1 : InportShadow  Port=2
  I2 : InportShadow  Port=2
  Sum1 : Sum  Inputs=-+|
  Sum2 : Sum  Inputs=|++
  Sum3 : Sum  Inputs=+-|
  Switch : Switch  Criteria=u2 ~= 0  SaturateOnIntegerOverflow=off  InputSameDT=off
  Unit Delay : UnitDelay  SampleTime=-1  HasFrameUpgradeWarning=on
  Vout : Outport  VectorParamsAs1DForOutWhenUnconnected=off
  wires:
  Compare To Zero/1 -> Switch/2
  I/1 -> Gain/1
  Constant/1 -> Sum2/2
  Sum2/1 -> Switch/1
  Unit Delay/1 -> Vout/1
  Gain/1 -> Sum2/1
  Vin/1 -> Sum3/1
  Switch/1 -> Sum3/2
  Gain1/1 -> Sum1/2
  Constant1/1 -> Sum1/1
  I2/1 -> Gain1/1
  Sum1/1 -> Switch/3
  Sum3/1 -> Unit Delay/1
  I1/1 -> Compare To Zero/1

== system slrt2levelinverterlib/Subcycle Averaging 2-Level Inverter /Half-Bridge SCA Math A/Short Between Rails Characteristics ==
  Vpos : Inport
  Vneg : Inport  Port=2
  Gain : Gain  Gain=1/2
  Subtract : Sum  Inputs=+-
  Unit Delay3 : UnitDelay  SampleTime=-1  HasFrameUpgradeWarning=on
  Out1 : Outport
  wires:
  Gain/1 -> Unit Delay3/1
  Subtract/1 -> Gain/1
  Vneg/1 -> Subtract/2
  Unit Delay3/1 -> Out1/1
  Vpos/1 -> Subtract/1

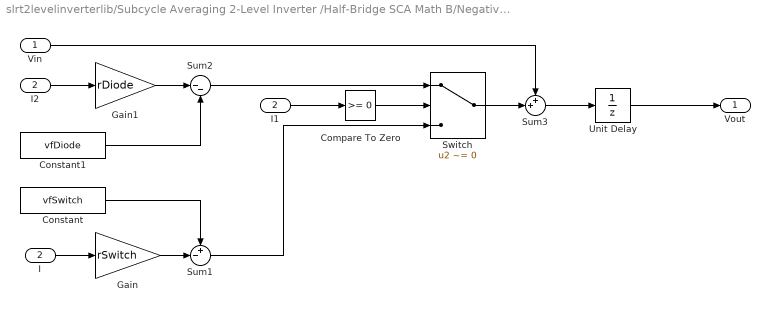
== system slrt2levelinverterlib/Subcycle Averaging 2-Level Inverter /Half-Bridge SCA Math B/Negative Rail Switch Characteristics ==
  Vin : Inport
  I : Inport  Port=2
  Compare To Zero : simulink/Logic and Bit Operations/Compare To Zero  relop=>=  OutDataTypeStr=boolean
  Constant : Constant  Value=vfSwitch  OutDataTypeStr=single  SampleTime=ts_Model
  Constant1 : Constant  Value=vfDiode  OutDataTypeStr=single  SampleTime=ts_Model
  Gain : Gain  Gain=rSwitch
  Gain1 : Gain  Gain=rDiode
  I1 : InportShadow  Port=2
  I2 : InportShadow  Port=2
  Sum1 : Sum  Inputs=+-|
  Sum2 : Sum  Inputs=|--
  Sum3 : Sum  Inputs=++|
  Switch : Switch  Criteria=u2 ~= 0  SaturateOnIntegerOverflow=off  InputSameDT=off
  Unit Delay : UnitDelay  SampleTime=-1  HasFrameUpgradeWarning=on
  Vout : Outport  VectorParamsAs1DForOutWhenUnconnected=off
  wires:
  I/1 -> Gain/1
  Gain1/1 -> Sum2/1
  Sum3/1 -> Unit Delay/1
  Switch/1 -> Sum3/2
  I1/1 -> Compare To Zero/1
  Vin/1 -> Sum3/1
  Unit Delay/1 -> Vout/1
  Constant/1 -> Sum1/1
  I2/1 -> Gain1/1
  Sum1/1 -> Switch/3
  Gain/1 -> Sum1/2
  Sum2/1 -> Switch/1
  Constant1/1 -> Sum2/2
  Compare To Zero/1 -> Switch/2

== system slrt2levelinverterlib/Subcycle Averaging 2-Level Inverter /Half-Bridge SCA Math B/Open Circuit ==
  + : Inport
  In : Inport  Port=2
  - : Inport  Port=3
  Gain : Gain  Gain=-rSnub
  Max : MinMax  Inputs=2
  Max1 : MinMax  Function=max  Inputs=2
  Unit Delay : UnitDelay  SampleTime=-1  HasFrameUpgradeWarning=on
  Out : Outport  VectorParamsAs1DForOutWhenUnconnected=off
  wires:
  -/1 -> Max1/2
  Max/1 -> Unit Delay/1
  +/1 -> Max/1
  Gain/1 -> Max1/1
  In/1 -> Gain/1
  Max1/1 -> Max/2
  Unit Delay/1 -> Out/1

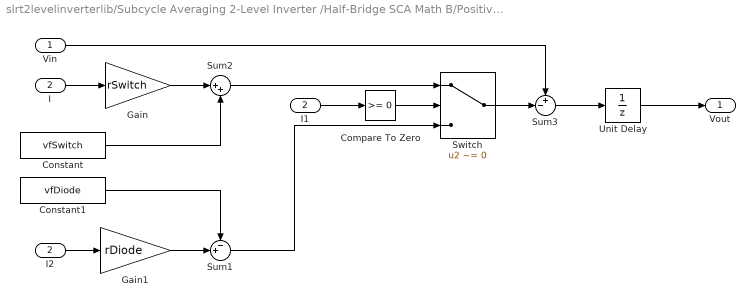
== system slrt2levelinverterlib/Subcycle Averaging 2-Level Inverter /Half-Bridge SCA Math B/Positive Rail Switch Characteristics ==
  Vin : Inport
  I : Inport  Port=2
  Compare To Zero : simulink/Logic and Bit Operations/Compare To Zero  relop=>=  OutDataTypeStr=boolean
  Constant : Constant  Value=vfSwitch  OutDataTypeStr=single  SampleTime=ts_Model
  Constant1 : Constant  Value=vfDiode  OutDataTypeStr=single  SampleTime=ts_Model
  Gain : Gain  Gain=rSwitch
  Gain1 : Gain  Gain=rDiode
  I1 : InportShadow  Port=2
  I2 : InportShadow  Port=2
  Sum1 : Sum  Inputs=-+|
  Sum2 : Sum  Inputs=|++
  Sum3 : Sum  Inputs=+-|
  Switch : Switch  Criteria=u2 ~= 0  SaturateOnIntegerOverflow=off  InputSameDT=off
  Unit Delay : UnitDelay  SampleTime=-1  HasFrameUpgradeWarning=on
  Vout : Outport  VectorParamsAs1DForOutWhenUnconnected=off
  wires:
  Compare To Zero/1 -> Switch/2
  I/1 -> Gain/1
  Constant/1 -> Sum2/2
  Sum2/1 -> Switch/1
  Unit Delay/1 -> Vout/1
  Gain/1 -> Sum2/1
  Vin/1 -> Sum3/1
  Switch/1 -> Sum3/2
  Gain1/1 -> Sum1/2
  Constant1/1 -> Sum1/1
  I2/1 -> Gain1/1
  Sum1/1 -> Switch/3
  Sum3/1 -> Unit Delay/1
  I1/1 -> Compare To Zero/1

== system slrt2levelinverterlib/Subcycle Averaging 2-Level Inverter /Half-Bridge SCA Math B/Short Between Rails Characteristics ==
  Vpos : Inport
  Vneg : Inport  Port=2
  Gain : Gain  Gain=1/2
  Subtract : Sum  Inputs=+-
  Unit Delay3 : UnitDelay  SampleTime=-1  HasFrameUpgradeWarning=on
  Out1 : Outport
  wires:
  Gain/1 -> Unit Delay3/1
  Subtract/1 -> Gain/1
  Vneg/1 -> Subtract/2
  Unit Delay3/1 -> Out1/1
  Vpos/1 -> Subtract/1

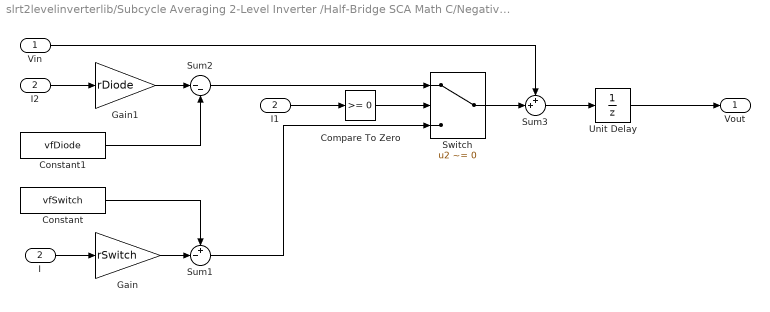
== system slrt2levelinverterlib/Subcycle Averaging 2-Level Inverter /Half-Bridge SCA Math C/Negative Rail Switch Characteristics ==
  Vin : Inport
  I : Inport  Port=2
  Compare To Zero : simulink/Logic and Bit Operations/Compare To Zero  relop=>=  OutDataTypeStr=boolean
  Constant : Constant  Value=vfSwitch  OutDataTypeStr=single  SampleTime=ts_Model
  Constant1 : Constant  Value=vfDiode  OutDataTypeStr=single  SampleTime=ts_Model
  Gain : Gain  Gain=rSwitch
  Gain1 : Gain  Gain=rDiode
  I1 : InportShadow  Port=2
  I2 : InportShadow  Port=2
  Sum1 : Sum  Inputs=+-|
  Sum2 : Sum  Inputs=|--
  Sum3 : Sum  Inputs=++|
  Switch : Switch  Criteria=u2 ~= 0  SaturateOnIntegerOverflow=off  InputSameDT=off
  Unit Delay : UnitDelay  SampleTime=-1  HasFrameUpgradeWarning=on
  Vout : Outport  VectorParamsAs1DForOutWhenUnconnected=off
  wires:
  I/1 -> Gain/1
  Gain1/1 -> Sum2/1
  Sum3/1 -> Unit Delay/1
  Switch/1 -> Sum3/2
  I1/1 -> Compare To Zero/1
  Vin/1 -> Sum3/1
  Unit Delay/1 -> Vout/1
  Constant/1 -> Sum1/1
  I2/1 -> Gain1/1
  Sum1/1 -> Switch/3
  Gain/1 -> Sum1/2
  Sum2/1 -> Switch/1
  Constant1/1 -> Sum2/2
  Compare To Zero/1 -> Switch/2

== system slrt2levelinverterlib/Subcycle Averaging 2-Level Inverter /Half-Bridge SCA Math C/Open Circuit ==
  + : Inport
  In : Inport  Port=2
  - : Inport  Port=3
  Gain : Gain  Gain=-rSnub
  Max : MinMax  Inputs=2
  Max1 : MinMax  Function=max  Inputs=2
  Unit Delay : UnitDelay  SampleTime=-1  HasFrameUpgradeWarning=on
  Out : Outport  VectorParamsAs1DForOutWhenUnconnected=off
  wires:
  -/1 -> Max1/2
  Max/1 -> Unit Delay/1
  +/1 -> Max/1
  Gain/1 -> Max1/1
  In/1 -> Gain/1
  Max1/1 -> Max/2
  Unit Delay/1 -> Out/1

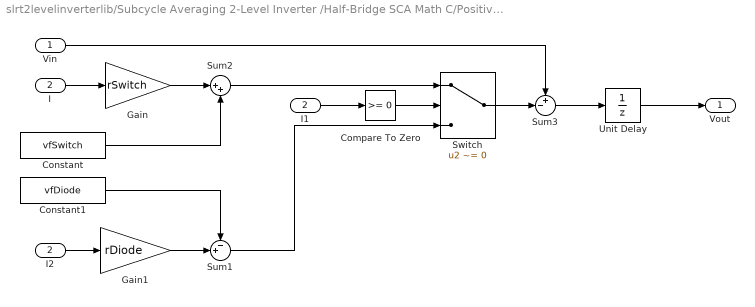
== system slrt2levelinverterlib/Subcycle Averaging 2-Level Inverter /Half-Bridge SCA Math C/Positive Rail Switch Characteristics ==
  Vin : Inport
  I : Inport  Port=2
  Compare To Zero : simulink/Logic and Bit Operations/Compare To Zero  relop=>=  OutDataTypeStr=boolean
  Constant : Constant  Value=vfSwitch  OutDataTypeStr=single  SampleTime=ts_Model
  Constant1 : Constant  Value=vfDiode  OutDataTypeStr=single  SampleTime=ts_Model
  Gain : Gain  Gain=rSwitch
  Gain1 : Gain  Gain=rDiode
  I1 : InportShadow  Port=2
  I2 : InportShadow  Port=2
  Sum1 : Sum  Inputs=-+|
  Sum2 : Sum  Inputs=|++
  Sum3 : Sum  Inputs=+-|
  Switch : Switch  Criteria=u2 ~= 0  SaturateOnIntegerOverflow=off  InputSameDT=off
  Unit Delay : UnitDelay  SampleTime=-1  HasFrameUpgradeWarning=on
  Vout : Outport  VectorParamsAs1DForOutWhenUnconnected=off
  wires:
  Compare To Zero/1 -> Switch/2
  I/1 -> Gain/1
  Constant/1 -> Sum2/2
  Sum2/1 -> Switch/1
  Unit Delay/1 -> Vout/1
  Gain/1 -> Sum2/1
  Vin/1 -> Sum3/1
  Switch/1 -> Sum3/2
  Gain1/1 -> Sum1/2
  Constant1/1 -> Sum1/1
  I2/1 -> Gain1/1
  Sum1/1 -> Switch/3
  Sum3/1 -> Unit Delay/1
  I1/1 -> Compare To Zero/1

== system slrt2levelinverterlib/Subcycle Averaging 2-Level Inverter /Half-Bridge SCA Math C/Short Between Rails Characteristics ==
  Vpos : Inport
  Vneg : Inport  Port=2
  Gain : Gain  Gain=1/2
  Subtract : Sum  Inputs=+-
  Unit Delay3 : UnitDelay  SampleTime=-1  HasFrameUpgradeWarning=on
  Out1 : Outport
  wires:
  Gain/1 -> Unit Delay3/1
  Subtract/1 -> Gain/1
  Vneg/1 -> Subtract/2
  Unit Delay3/1 -> Out1/1
  Vpos/1 -> Subtract/1
